simulink model "multilevel"  (R2018b)
settings: Solver=VariableStepAuto  StartTime=0.0  StopTime=10  RelTol=1e-3
undefined symbols (not defined in the file): Ion, Lithium
libraries: powerlib x23, simulink x3, electricdrivelib x1
settings Model: Creator=user  LastModifiedBy=user

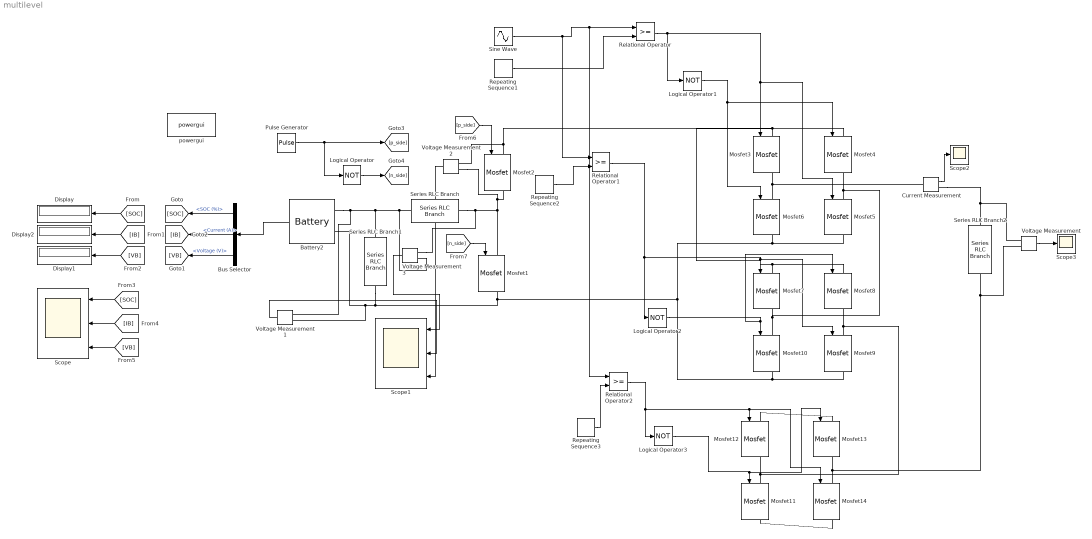
== system multilevel ==
  Battery2 : electricdrivelib/Extra Sources/Battery  BatType=Lithium-Ion  ShowTempParam=off  ThermalPreset=no  ShowAgeParam=off  NomV=24  NomQ=10  SOC=50  Batt_Tr=1e-4  PresetModel=on  MaxQ=10  MinV=18  FullV=27.9357  Dis_rate=4.3478  R=0.024  Normal_OP=9.0435  expZone="[25.9293     0.491304]"  current=[6.5 13 32.5]  Units=Time  Tci=20  NomT=20  T2=-30  MaxQ2=4.8  FullV2=7.1  Normal_OP2=5.655  expZone2="[6.58           1]"  Rca=0.6  ti=2000  Dp=0  Neq0=0  Tsim=1e6  Ta1=25  Qeol=5.4*0.9  Reol=0.013333*1.2  Char_age=[2.3478, 3]  Dis_age=[2.3478, 10]  N1=1500  N2=10500  N3=1000  N4=1400  Ta2=45  N5=950
  Bus Selector : BusSelector  OutputSignals=SOC (%),Current (A),Voltage (V)
  Current Measurement : powerlib/Measurements/Current Measurement  PhasorSimulation=off  OutputType=Complex  PSBequivalent=0
  Display : Display
  Display1 : Display
  Display2 : Display
  Logical Operator : Logic  Operator=NOT  AllPortsSameDT=off  OutDataTypeStr=boolean
  Logical Operator1 : Logic  Operator=NOT  IconShape=distinctive  AllPortsSameDT=off  OutDataTypeStr=boolean
  Logical Operator2 : Logic  Operator=NOT  IconShape=distinctive  AllPortsSameDT=off  OutDataTypeStr=boolean
  Logical Operator3 : Logic  Operator=NOT  IconShape=distinctive  AllPortsSameDT=off  OutDataTypeStr=boolean
  Mosfet{1..14} (14 alike) : powerlib/Power Electronics/Mosfet  Ron=0.1  Lon=0  Rd=0.01  Vfd=0  IC=0  Rs=1e5  Cs=inf  Measurements=on
  Pulse Generator : DiscretePulseGenerator  PulseType=Time based  Period=1e-4  PulseWidth=40
  Relational Operator : RelationalOperator  OutDataTypeStr=boolean  RndMeth=Simplest
  Relational Operator1 : RelationalOperator  OutDataTypeStr=boolean  RndMeth=Simplest
  Relational Operator2 : RelationalOperator  OutDataTypeStr=boolean  RndMeth=Simplest
  Repeating Sequence1 : simulink/Sources/Repeating Sequence  rep_seq_t=[0 1]  rep_seq_y=[0 1]
  Repeating Sequence2 : simulink/Sources/Repeating Sequence  rep_seq_t=[0 1]  rep_seq_y=[1 2]
  Repeating Sequence3 : simulink/Sources/Repeating Sequence  rep_seq_t=[0 1]  rep_seq_y=[2 3]
  Scope : Scope  NumInputPorts=3
  Scope1 : Scope  NumInputPorts=3
  Scope2 : Scope
  Scope3 : Scope
  Series RLC Branch : powerlib/Elements/Series RLC Branch  LConnTagsString=__new0  RConnTagsString=__new0  BranchType=RL  Resistance=0.1  Inductance=1e-3  SetiL0=off  InitialCurrent=0  Capacitance=1e-6  Setx0=off  InitialVoltage=0  Measurements=None
  Series RLC Branch1 : powerlib/Elements/Series RLC Branch  LConnTagsString=__new0  RConnTagsString=__new0  BranchType=RC  Resistance=0.1  Inductance=1e-3  SetiL0=off  InitialCurrent=0  Capacitance=1e-6  Setx0=off  InitialVoltage=0  Measurements=None
  Series RLC Branch2 : powerlib/Elements/Series RLC Branch  LConnTagsString=__new0  RConnTagsString=__new0  BranchType=R  Resistance=1  Inductance=1e-3  SetiL0=off  InitialCurrent=0  Capacitance=1e-6  Setx0=off  InitialVoltage=0  Measurements=None
  Sine Wave : Sin  Amplitude=3  Frequency=2*pi*50  SampleTime=0
  Voltage Measurement{,1..3} (4 alike) : powerlib/Measurements/Voltage Measurement  PhasorSimulation=off  OutputType=Complex  PSBequivalent=0
  powergui : powerlib/powergui  Priority=1  SimulationMode=Discrete  SampleTime=50e-6  frequency=60  Iterations=50  frequencyindice=0  Pbase=100e6  ErrMax=1e-4  UnitsV=kV  UnitsW=MW  buscounter=0  FunctionMessages=off  echomessages=off  EnableUseOfTLC=off  CurrentSourceSwitches=off  DisableSnubberDevices=off  DisableRonSwitches=off  DisableVfSwitches=off  DisplayEquations=off  SolverType=Tustin/Backward Euler (TBE)  Interpol=off  ExternalGateDelay=off  methode=off  Ts=100  x0status=blocks  SPID=on  SwTol=0  HookPort=off  RestoreLinks=warning  ResistiveCurrentMeasurement=off  Frange=[0:2:500]  Ylog=off  Xlog=on  ShowGrid=off  save=off  variable=ZData  structure=volt  ZoomFFT=off  StartTime=1  cycles=5  DisplayStyle=1  fundamental=50  FreqAxis=off  MaxFrequency=250  frequencyindicesteady=1  RmsSteady=1  display=off
  wires:
  [SOC] -> Display/1
  Logical Operator/1 -> [n_side]
  [n_side] -> Mosfet1/1
  Battery2/1 -> Bus Selector/1
  Voltage Measurement1/1 -> Scope1/2
  [IB] -> Scope/2
  [VB] -> Scope/3
  Voltage Measurement3/1 -> Scope1/1
  Pulse Generator/1 -> Logical Operator/1, [p_side]
  Bus Selector/1 -> [SOC]  "<SOC (%)>"
  Bus Selector/3 -> [VB]  "<Voltage (V)>"
  [VB] -> Display1/1
  Bus Selector/2 -> [IB]  "<Current (A)>"
  [p_side] -> Mosfet2/1
  [SOC] -> Scope/1
  [IB] -> Display2/1
  Voltage Measurement2/1 -> Scope1/3
  Current Measurement/1 -> Scope2/1
  Sine Wave/1 -> Relational Operator1/1, Relational Operator2/1, Relational Operator/1
  Repeating Sequence1/1 -> Relational Operator/2
  Relational Operator/1 -> Logical Operator1/1, Mosfet5/1, Mosfet3/1
  Logical Operator1/1 -> Mosfet4/1, Mosfet6/1
  Repeating Sequence2/1 -> Relational Operator1/2
  Relational Operator1/1 -> Logical Operator2/1, Mosfet9/1, Mosfet7/1
  Logical Operator2/1 -> Mosfet8/1, Mosfet10/1
  Voltage Measurement/1 -> Scope3/1
  Repeating Sequence3/1 -> Relational Operator2/2
  Relational Operator2/1 -> Logical Operator3/1, Mosfet14/1, Mosfet12/1
  Logical Operator3/1 -> Mosfet13/1, Mosfet11/1
  connections:
  Series RLC Branch/RConn1 -- Voltage Measurement1/LConn1 -- Battery2/LConn1 -- Series RLC Branch1/LConn1 -- Voltage Measurement3/LConn2
  Mosfet2/RConn1 -- Voltage Measurement2/LConn2 -- Voltage Measurement3/LConn1 -- Series RLC Branch/LConn1 -- Mosfet1/LConn1
  Mosfet6/LConn1 -- Mosfet3/RConn1 -- Current Measurement/LConn1
  Series RLC Branch1/RConn1 -- Voltage Measurement1/LConn2 -- Battery2/LConn2 -- Mosfet5/RConn1 -- Mosfet6/RConn1 -- Mosfet9/RConn1 -- Mosfet10/RConn1 -- Mosfet1/RConn1
  Mosfet2/LConn1 -- Mosfet4/LConn1 -- Mosfet3/LConn1 -- Mosfet8/LConn1 -- Mosfet7/LConn1 -- Voltage Measurement2/LConn1
  Current Measurement/RConn1 -- Voltage Measurement/LConn1 -- Series RLC Branch2/LConn1
  Mosfet14/RConn1 -- Mosfet11/RConn1
  Mosfet12/LConn1 -- Mosfet13/LConn1
  Mosfet5/LConn1 -- Mosfet10/LConn1 -- Mosfet7/RConn1 -- Mosfet4/RConn1
  Voltage Measurement/LConn2 -- Mosfet13/RConn1 -- Mosfet14/LConn1 -- Series RLC Branch2/RConn1
  Mosfet11/LConn1 -- Mosfet9/LConn1 -- Mosfet8/RConn1 -- Mosfet12/RConn1
